simulink model "gm_final_heart_sym2_level4_hdl"  (R2021a)
settings: Solver=FixedStepDiscrete  StartTime=0.0  StopTime=8  RelTol=1e-3
libraries: hdlmdlgenlib x45
(part 3 of 3)

== system gm_final_heart_sym2_level4_hdl/DWT_Sym2_Level4/1st_Level_Recon2/LoR_Odd ==
  In_LoR_o : Inport  OutDataTypeStr=fixdt(1, 16, 23)  PortDimensions=1  SampleTime=2.26757369614512e-05
  Add : Sum  AccumDataTypeStr=fixdt(1, 16, 23)  OutDataTypeStr=fixdt(1, 16, 23)  SampleTime=2.26757369614512e-05
  Constant11 : Constant  Value=-0.1294097900390625  OutDataTypeStr=fixdt(1, 16, 17)  SampleTime=2.26757369614512e-05
  Constant9 : Constant  Value=0.836517333984375  OutDataTypeStr=fixdt(0, 16, 16)  SampleTime=2.26757369614512e-05
  Delay : Delay  DelayLength=double(1)  InitialCondition=0  SampleTime=2.26757369614512e-05
  HwModeRegister{,1..3} (4 alike) : Delay  DelayLength=double(1)  InitialCondition=0  SampleTime=2.26757369614512e-05
  Multiply : Product  Inputs=**  OutDataTypeStr=fixdt(1, 16, 23)  SampleTime=2.26757369614512e-05
  Multiply1 : Product  Inputs=**  OutDataTypeStr=fixdt(1, 16, 26)  SampleTime=2.26757369614512e-05
  PipelineRegister : Delay  DelayLength=double(1)  InitialCondition=0  SampleTime=2.26757369614512e-05
  PipelineRegister1 : Delay  DelayLength=double(1)  InitialCondition=0  SampleTime=2.26757369614512e-05
  Rate Transition : hdlmdlgenlib/Buffer
      settings: SourceProductBaseCode=SL
  delayMatch : Delay  DelayLength=double(1)  InitialCondition=0  SampleTime=2.26757369614512e-05
  Out_HiR_o : Outport  OutDataTypeStr=fixdt(1,16,23)  SampleTime=2.26757369614512e-05  VectorParamsAs1DForOutWhenUnconnected=off
  wires:
  Add/1 -> Out_HiR_o/1
  Constant11/1 -> HwModeRegister2/1
  Constant9/1 -> HwModeRegister/1
  Delay/1 -> Rate Transition/1
  PipelineRegister/1 -> Add/1
  delayMatch/1 -> Add/2
  Rate Transition/1 -> HwModeRegister3/1
  In_LoR_o/1 -> Delay/1, HwModeRegister1/1
  PipelineRegister1/1 -> delayMatch/1
  Multiply/1 -> PipelineRegister/1
  HwModeRegister/1 -> Multiply/1
  HwModeRegister1/1 -> Multiply/2
  Multiply1/1 -> PipelineRegister1/1
  HwModeRegister2/1 -> Multiply1/1
  HwModeRegister3/1 -> Multiply1/2

== system gm_final_heart_sym2_level4_hdl/DWT_Sym2_Level4/1st_Level_Recon3/HiR_Even ==
  In_HiR_e : Inport  OutDataTypeStr=fixdt(1, 16, 28)  PortDimensions=1  SampleTime=2.26757369614512e-05
  Add : Sum  AccumDataTypeStr=fixdt(1, 16, 28)  OutDataTypeStr=fixdt(1, 16, 28)  SampleTime=2.26757369614512e-05
  Constant12 : Constant  Value=-0.1294097900390625  OutDataTypeStr=fixdt(1, 16, 17)  SampleTime=2.26757369614512e-05
  Constant14 : Constant  Value=0.836517333984375  OutDataTypeStr=fixdt(0, 16, 16)  SampleTime=2.26757369614512e-05
  Delay : Delay  DelayLength=double(1)  InitialCondition=0  SampleTime=2.26757369614512e-05
  HwModeRegister{,1..3} (4 alike) : Delay  DelayLength=double(1)  InitialCondition=0  SampleTime=2.26757369614512e-05
  Multiply : Product  Inputs=**  OutDataTypeStr=fixdt(1, 16, 30)  SampleTime=2.26757369614512e-05
  Multiply1 : Product  Inputs=**  OutDataTypeStr=fixdt(1, 16, 28)  SampleTime=2.26757369614512e-05
  PipelineRegister : Delay  DelayLength=double(1)  InitialCondition=0  SampleTime=2.26757369614512e-05
  PipelineRegister1 : Delay  DelayLength=double(1)  InitialCondition=0  SampleTime=2.26757369614512e-05
  Rate Transition : hdlmdlgenlib/Buffer
      settings: SourceProductBaseCode=SL
  delayMatch : Delay  DelayLength=double(1)  InitialCondition=0  SampleTime=2.26757369614512e-05
  Out_HiR_e : Outport  OutDataTypeStr=fixdt(1,16,28)  SampleTime=2.26757369614512e-05  VectorParamsAs1DForOutWhenUnconnected=off
  wires:
  Add/1 -> Out_HiR_e/1
  Constant12/1 -> HwModeRegister/1
  Constant14/1 -> HwModeRegister2/1
  Delay/1 -> Rate Transition/1
  PipelineRegister/1 -> Add/1
  delayMatch/1 -> Add/2
  Rate Transition/1 -> HwModeRegister3/1
  In_HiR_e/1 -> Delay/1, HwModeRegister1/1
  PipelineRegister1/1 -> delayMatch/1
  Multiply/1 -> PipelineRegister/1
  HwModeRegister/1 -> Multiply/1
  HwModeRegister1/1 -> Multiply/2
  Multiply1/1 -> PipelineRegister1/1
  HwModeRegister2/1 -> Multiply1/1
  HwModeRegister3/1 -> Multiply1/2

== system gm_final_heart_sym2_level4_hdl/DWT_Sym2_Level4/1st_Level_Recon3/HiR_Odd ==
  In_HiR_o : Inport  OutDataTypeStr=fixdt(1, 16, 28)  PortDimensions=1  SampleTime=2.26757369614512e-05
  Add : Sum  AccumDataTypeStr=fixdt(1, 16, 28)  OutDataTypeStr=fixdt(1, 16, 28)  SampleTime=2.26757369614512e-05
  Constant13 : Constant  Value=-0.22414398193359375  OutDataTypeStr=fixdt(1, 16, 17)  SampleTime=2.26757369614512e-05
  Constant15 : Constant  Value=-0.4829559326171875  OutDataTypeStr=fixdt(1, 16, 16)  SampleTime=2.26757369614512e-05
  Delay : Delay  DelayLength=double(1)  InitialCondition=0  SampleTime=2.26757369614512e-05
  HwModeRegister{,1..3} (4 alike) : Delay  DelayLength=double(1)  InitialCondition=0  SampleTime=2.26757369614512e-05
  Multiply : Product  Inputs=**  OutDataTypeStr=fixdt(1, 16, 30)  SampleTime=2.26757369614512e-05
  Multiply1 : Product  Inputs=**  OutDataTypeStr=fixdt(1, 16, 29)  SampleTime=2.26757369614512e-05
  PipelineRegister : Delay  DelayLength=double(1)  InitialCondition=0  SampleTime=2.26757369614512e-05
  PipelineRegister1 : Delay  DelayLength=double(1)  InitialCondition=0  SampleTime=2.26757369614512e-05
  Rate Transition : hdlmdlgenlib/Buffer
      settings: SourceProductBaseCode=SL
  delayMatch : Delay  DelayLength=double(1)  InitialCondition=0  SampleTime=2.26757369614512e-05
  Out_HiR_o : Outport  OutDataTypeStr=fixdt(1,16,28)  SampleTime=2.26757369614512e-05  VectorParamsAs1DForOutWhenUnconnected=off
  wires:
  Add/1 -> Out_HiR_o/1
  Constant13/1 -> HwModeRegister/1
  Constant15/1 -> HwModeRegister2/1
  Delay/1 -> Rate Transition/1
  PipelineRegister/1 -> Add/1
  delayMatch/1 -> Add/2
  Rate Transition/1 -> HwModeRegister3/1
  In_HiR_o/1 -> Delay/1, HwModeRegister1/1
  PipelineRegister1/1 -> delayMatch/1
  Multiply/1 -> PipelineRegister/1
  HwModeRegister/1 -> Multiply/1
  HwModeRegister1/1 -> Multiply/2
  Multiply1/1 -> PipelineRegister1/1
  HwModeRegister2/1 -> Multiply1/1
  HwModeRegister3/1 -> Multiply1/2

== system gm_final_heart_sym2_level4_hdl/DWT_Sym2_Level4/1st_Level_Recon3/LoR_Even ==
  In_LoR_e : Inport  OutDataTypeStr=fixdt(1, 16, 22)  PortDimensions=1  SampleTime=2.26757369614512e-05
  Add : Sum  AccumDataTypeStr=fixdt(1, 16, 23)  OutDataTypeStr=fixdt(1, 16, 23)  SampleTime=2.26757369614512e-05
  Constant10 : Constant  Value=0.22414398193359375  OutDataTypeStr=fixdt(0, 16, 18)  SampleTime=2.26757369614512e-05
  Constant8 : Constant  Value=0.48296356201171875  OutDataTypeStr=fixdt(0, 16, 17)  SampleTime=2.26757369614512e-05
  Delay : Delay  DelayLength=double(1)  InitialCondition=0  SampleTime=2.26757369614512e-05
  HwModeRegister{,1..3} (4 alike) : Delay  DelayLength=double(1)  InitialCondition=0  SampleTime=2.26757369614512e-05
  Multiply : Product  Inputs=**  OutDataTypeStr=fixdt(1, 16, 23)  SampleTime=2.26757369614512e-05
  Multiply1 : Product  Inputs=**  OutDataTypeStr=fixdt(1, 16, 25)  SampleTime=2.26757369614512e-05
  PipelineRegister : Delay  DelayLength=double(1)  InitialCondition=0  SampleTime=2.26757369614512e-05
  PipelineRegister1 : Delay  DelayLength=double(1)  InitialCondition=0  SampleTime=2.26757369614512e-05
  Rate Transition : hdlmdlgenlib/Buffer
      settings: SourceProductBaseCode=SL
  delayMatch : Delay  DelayLength=double(1)  InitialCondition=0  SampleTime=2.26757369614512e-05
  Out_LoR_e : Outport  OutDataTypeStr=fixdt(1,16,23)  SampleTime=2.26757369614512e-05  VectorParamsAs1DForOutWhenUnconnected=off
  wires:
  Add/1 -> Out_LoR_e/1
  Constant10/1 -> HwModeRegister2/1
  Constant8/1 -> HwModeRegister/1
  Delay/1 -> Rate Transition/1
  PipelineRegister/1 -> Add/1
  delayMatch/1 -> Add/2
  Rate Transition/1 -> HwModeRegister3/1
  In_LoR_e/1 -> Delay/1, HwModeRegister1/1
  PipelineRegister1/1 -> delayMatch/1
  Multiply/1 -> PipelineRegister/1
  HwModeRegister/1 -> Multiply/1
  HwModeRegister1/1 -> Multiply/2
  Multiply1/1 -> PipelineRegister1/1
  HwModeRegister2/1 -> Multiply1/1
  HwModeRegister3/1 -> Multiply1/2

== system gm_final_heart_sym2_level4_hdl/DWT_Sym2_Level4/1st_Level_Recon3/LoR_Odd ==
  In_LoR_o : Inport  OutDataTypeStr=fixdt(1, 16, 22)  PortDimensions=1  SampleTime=2.26757369614512e-05
  Add : Sum  AccumDataTypeStr=fixdt(1, 16, 23)  OutDataTypeStr=fixdt(1, 16, 23)  SampleTime=2.26757369614512e-05
  Constant11 : Constant  Value=-0.1294097900390625  OutDataTypeStr=fixdt(1, 16, 17)  SampleTime=2.26757369614512e-05
  Constant9 : Constant  Value=0.836517333984375  OutDataTypeStr=fixdt(0, 16, 16)  SampleTime=2.26757369614512e-05
  Delay : Delay  DelayLength=double(1)  InitialCondition=0  SampleTime=2.26757369614512e-05
  HwModeRegister{,1..3} (4 alike) : Delay  DelayLength=double(1)  InitialCondition=0  SampleTime=2.26757369614512e-05
  Multiply : Product  Inputs=**  OutDataTypeStr=fixdt(1, 16, 23)  SampleTime=2.26757369614512e-05
  Multiply1 : Product  Inputs=**  OutDataTypeStr=fixdt(1, 16, 25)  SampleTime=2.26757369614512e-05
  PipelineRegister : Delay  DelayLength=double(1)  InitialCondition=0  SampleTime=2.26757369614512e-05
  PipelineRegister1 : Delay  DelayLength=double(1)  InitialCondition=0  SampleTime=2.26757369614512e-05
  Rate Transition : hdlmdlgenlib/Buffer
      settings: SourceProductBaseCode=SL
  delayMatch : Delay  DelayLength=double(1)  InitialCondition=0  SampleTime=2.26757369614512e-05
  Out_HiR_o : Outport  OutDataTypeStr=fixdt(1,16,23)  SampleTime=2.26757369614512e-05  VectorParamsAs1DForOutWhenUnconnected=off
  wires:
  Add/1 -> Out_HiR_o/1
  Constant11/1 -> HwModeRegister2/1
  Constant9/1 -> HwModeRegister/1
  Delay/1 -> Rate Transition/1
  PipelineRegister/1 -> Add/1
  delayMatch/1 -> Add/2
  Rate Transition/1 -> HwModeRegister3/1
  In_LoR_o/1 -> Delay/1, HwModeRegister1/1
  PipelineRegister1/1 -> delayMatch/1
  Multiply/1 -> PipelineRegister/1
  HwModeRegister/1 -> Multiply/1
  HwModeRegister1/1 -> Multiply/2
  Multiply1/1 -> PipelineRegister1/1
  HwModeRegister2/1 -> Multiply1/1
  HwModeRegister3/1 -> Multiply1/2

== system gm_final_heart_sym2_level4_hdl/DWT_Sym2_Level4/Threshold_Estimator/Absolute_Value1 ==
  Signal_w4 : Inport  OutDataTypeStr=fixdt(1, 16, 26)  PortDimensions=1  SampleTime=2.26757369614512e-05
  Absolute_Switch : Switch  Threshold=double(1)  OutDataTypeStr=fixdt(0, 16, 27)  SampleTime=2.26757369614512e-05
  Constant295 : Constant  Value=0  OutDataTypeStr=fixdt(1, 16, 4)  SampleTime=2.26757369614512e-05
  Gain2 : Product  Inputs=**  OutDataTypeStr=fixdt(0, 16, 28)  SampleTime=2.26757369614512e-05
  Gain2_const : Constant  Value=-1  OutDataTypeStr=fixdt(1, 16, 15)  SampleTime=2.26757369614512e-05
  HwModeRegister : Delay  DelayLength=double(1)  InitialCondition=0  SampleTime=2.26757369614512e-05
  HwModeRegister1 : Delay  DelayLength=double(1)  InitialCondition=0  SampleTime=2.26757369614512e-05
  PipelineRegister : Delay  DelayLength=double(1)  InitialCondition=0  SampleTime=2.26757369614512e-05
  Relational Operator2 : RelationalOperator  Operator=<  OutDataTypeStr=boolean  SampleTime=2.26757369614512e-05  RndMeth=Nearest
  delayMatch : Delay  DelayLength=double(2)  InitialCondition=0  SampleTime=2.26757369614512e-05
  delayMatch1 : Delay  DelayLength=double(2)  InitialCondition=0  SampleTime=2.26757369614512e-05
  Out_Abs : Outport  OutDataTypeStr=fixdt(0,16,27)  SampleTime=2.26757369614512e-05  VectorParamsAs1DForOutWhenUnconnected=off
  wires:
  delayMatch1/1 -> Absolute_Switch/3
  Absolute_Switch/1 -> Out_Abs/1
  Constant295/1 -> Relational Operator2/2
  PipelineRegister/1 -> Absolute_Switch/1
  delayMatch/1 -> Absolute_Switch/2
  Gain2_const/1 -> HwModeRegister/1
  Signal_w4/1 -> delayMatch1/1, Relational Operator2/1, HwModeRegister1/1
  Relational Operator2/1 -> delayMatch/1
  Gain2/1 -> PipelineRegister/1
  HwModeRegister/1 -> Gain2/1
  HwModeRegister1/1 -> Gain2/2

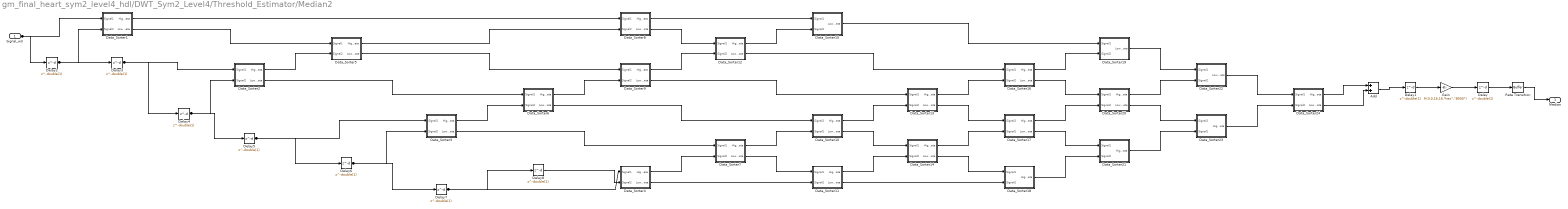
== system gm_final_heart_sym2_level4_hdl/DWT_Sym2_Level4/Threshold_Estimator/Median2 ==
  Signal_w3 : Inport  OutDataTypeStr=fixdt(0, 16, 27)  PortDimensions=1  SampleTime=2.26757369614512e-05
  Add : Sum  AccumDataTypeStr=fixdt(0, 16, 26)  OutDataTypeStr=fixdt(0, 16, 26)  SampleTime=2.26757369614512e-05
  Data_Sorter1 : Subsystem
  Data_Sorter10 : Subsystem
  Data_Sorter11 : Subsystem
  Data_Sorter12 : Subsystem
  Data_Sorter13 : Subsystem
  Data_Sorter14 : Subsystem
  Data_Sorter15 : Subsystem
  Data_Sorter16 : Subsystem
  Data_Sorter17 : Subsystem
  Data_Sorter18 : Subsystem
  Data_Sorter19 : Subsystem
  Data_Sorter2 : Subsystem
  Data_Sorter20 : Subsystem
  Data_Sorter21 : Subsystem
  Data_Sorter22 : Subsystem
  Data_Sorter23 : Subsystem
  Data_Sorter24 : Subsystem
  Data_Sorter3 : Subsystem
  Data_Sorter4 : Subsystem
  Data_Sorter5 : Subsystem
  Data_Sorter6 : Subsystem
  Data_Sorter7 : Subsystem
  Data_Sorter8 : Subsystem
  Data_Sorter9 : Subsystem
  Delay{,1..8} (9 alike) : Delay  DelayLength=double(1)  InitialCondition=0  SampleTime=2.26757369614512e-05
  Gain : Gain  Gain="fi(0,0,16,16,\"hex\",\"8000\")"  ParamDataTypeStr=fixdt(0, 16, 16)  OutDataTypeStr=fixdt(0, 16, 27)  SampleTime=2.26757369614512e-05
  Rate Transition : hdlmdlgenlib/Buffer
      settings: SourceProductBaseCode=SL
  Median : Outport  OutDataTypeStr=fixdt(0,16,27)  SampleTime=2.26757369614512e-05  VectorParamsAs1DForOutWhenUnconnected=off
  wires:
  Add/1 -> Delay1/1
  Data_Sorter1/1(High_Data) -> Data_Sorter8/1(Signal1)
  Data_Sorter1/2(Low_Data) -> Data_Sorter5/1(Signal1)
  Data_Sorter10/1(High_Data) -> Data_Sorter13/2(Signal2)
  Data_Sorter10/2(Low_Data) -> Data_Sorter14/1(Signal1)
  Data_Sorter11/1(High_Data) -> Data_Sorter14/2(Signal2)
  Data_Sorter11/2(Low_Data) -> Data_Sorter18/2(Signal2)
  Data_Sorter12/1(High_Data) -> Data_Sorter15/2(Signal2)
  Data_Sorter12/2(Low_Data) -> Data_Sorter16/1(Signal1)
  Data_Sorter13/1(High_Data) -> Data_Sorter16/2(Signal2)
  Data_Sorter13/2(Low_Data) -> Data_Sorter17/1(Signal1)
  Data_Sorter14/1(High_Data) -> Data_Sorter17/2(Signal2)
  Data_Sorter14/2(Low_Data) -> Data_Sorter18/1(Signal1)
  Data_Sorter15/1(Low_Data) -> Data_Sorter19/1(Signal1)
  Data_Sorter16/1(High_Data) -> Data_Sorter19/2(Signal2)
  Data_Sorter16/2(Low_Data) -> Data_Sorter20/1(Signal1)
  Data_Sorter17/1(High_Data) -> Data_Sorter20/2(Signal2)
  Data_Sorter17/2(Low_Data) -> Data_Sorter21/1(Signal1)
  Data_Sorter18/1(High_Data) -> Data_Sorter21/2(Signal2)
  Data_Sorter19/1(Low_Data) -> Data_Sorter22/1(Signal1)
  Data_Sorter2/1(High_Data) -> Data_Sorter5/2(Signal2)
  Data_Sorter2/2(Low_Data) -> Data_Sorter6/1(Signal1)
  Data_Sorter20/1(High_Data) -> Data_Sorter22/2(Signal2)
  Data_Sorter20/2(Low_Data) -> Data_Sorter23/1(Signal1)
  Data_Sorter21/1(High_Data) -> Data_Sorter23/2(Signal2)
  Data_Sorter22/1(Low_Data) -> Data_Sorter24/1(Signal1)
  Data_Sorter23/1(High_Data) -> Data_Sorter24/2(Signal2)
  Data_Sorter24/1(High_Data) -> Add/1
  Data_Sorter24/2(Low_Data) -> Add/2
  Data_Sorter3/1(High_Data) -> Data_Sorter6/2(Signal2)
  Data_Sorter3/2(Low_Data) -> Data_Sorter7/1(Signal1)
  Data_Sorter4/1(High_Data) -> Data_Sorter7/2(Signal2)
  Data_Sorter4/2(Low_Data) -> Data_Sorter11/2(Signal2)
  Data_Sorter5/1(High_Data) -> Data_Sorter8/2(Signal2)
  Data_Sorter5/2(Low_Data) -> Data_Sorter9/1(Signal1)
  Data_Sorter6/1(High_Data) -> Data_Sorter9/2(Signal2)
  Data_Sorter6/2(Low_Data) -> Data_Sorter10/1(Signal1)
  Data_Sorter7/1(High_Data) -> Data_Sorter10/2(Signal2)
  Data_Sorter7/2(Low_Data) -> Data_Sorter11/1(Signal1)
  Data_Sorter8/1(High_Data) -> Data_Sorter15/1(Signal1)
  Data_Sorter8/2(Low_Data) -> Data_Sorter12/1(Signal1)
  Data_Sorter9/1(High_Data) -> Data_Sorter12/2(Signal2)
  Data_Sorter9/2(Low_Data) -> Data_Sorter13/1(Signal1)
  Delay/1 -> Rate Transition/1
  Delay1/1 -> Gain/1
  Delay2/1 -> Delay3/1, Data_Sorter1/2(Signal2)
  Delay3/1 -> Delay4/1, Data_Sorter2/1(Signal1)
  Delay4/1 -> Delay5/1, Data_Sorter2/2(Signal2)
  Delay5/1 -> Delay6/1, Data_Sorter3/1(Signal1)
  Delay6/1 -> Delay7/1, Data_Sorter3/2(Signal2)
  Delay7/1 -> Delay8/1, Data_Sorter4/1(Signal1)
  Delay8/1 -> Data_Sorter4/2(Signal2)
  Gain/1 -> Delay/1
  Rate Transition/1 -> Median/1
  Signal_w3/1 -> Delay2/1, Data_Sorter1/1(Signal1)

== system gm_final_heart_sym2_level4_hdl/DWT_Sym2_Level4/Threshold_Estimator/Median2/Data_Sorter1 ==
  Signal1 : Inport  OutDataTypeStr=fixdt(0, 16, 27)  PortDimensions=1  SampleTime=2.26757369614512e-05
  Signal2 : Inport  Port=2  OutDataTypeStr=fixdt(0, 16, 27)  PortDimensions=1  SampleTime=2.26757369614512e-05
  Data_Sorter_Switch : Switch  Criteria=u2 ~= 0  Threshold=double(0)  OutDataTypeStr=fixdt(0, 16, 27)  SampleTime=2.26757369614512e-05
  Data_Sorter_Switch1 : Switch  Threshold=double(1)  OutDataTypeStr=fixdt(0, 16, 27)  SampleTime=2.26757369614512e-05
  Delay1 : Delay  DelayLength=double(1)  InitialCondition=0  SampleTime=2.26757369614512e-05
  Delay2 : Delay  DelayLength=double(1)  InitialCondition=0  SampleTime=2.26757369614512e-05
  Relational Operator2 : RelationalOperator  Operator=<  OutDataTypeStr=boolean  SampleTime=2.26757369614512e-05  RndMeth=Nearest
  High_Data : Outport  OutDataTypeStr=fixdt(0,16,27)  SampleTime=2.26757369614512e-05  VectorParamsAs1DForOutWhenUnconnected=off
  Low_Data : Outport  Port=2  OutDataTypeStr=fixdt(0,16,27)  SampleTime=2.26757369614512e-05  VectorParamsAs1DForOutWhenUnconnected=off
  wires:
  Data_Sorter_Switch/1 -> Delay1/1
  Data_Sorter_Switch1/1 -> Delay2/1
  Delay1/1 -> High_Data/1
  Delay2/1 -> Low_Data/1
  Relational Operator2/1 -> Data_Sorter_Switch1/2, Data_Sorter_Switch/2
  Signal1/1 -> Relational Operator2/1, Data_Sorter_Switch/3, Data_Sorter_Switch/1
  Signal2/1 -> Relational Operator2/2, Data_Sorter_Switch1/3, Data_Sorter_Switch1/1

== system gm_final_heart_sym2_level4_hdl/DWT_Sym2_Level4/Threshold_Estimator/Median2/Data_Sorter10 ==
  Signal1 : Inport  OutDataTypeStr=fixdt(0, 16, 27)  PortDimensions=1  SampleTime=2.26757369614512e-05
  Signal2 : Inport  Port=2  OutDataTypeStr=fixdt(0, 16, 27)  PortDimensions=1  SampleTime=2.26757369614512e-05
  Data_Sorter_Switch : Switch  Criteria=u2 ~= 0  Threshold=double(0)  OutDataTypeStr=fixdt(0, 16, 27)  SampleTime=2.26757369614512e-05
  Data_Sorter_Switch1 : Switch  Threshold=double(1)  OutDataTypeStr=fixdt(0, 16, 27)  SampleTime=2.26757369614512e-05
  Delay1 : Delay  DelayLength=double(1)  InitialCondition=0  SampleTime=2.26757369614512e-05
  Delay2 : Delay  DelayLength=double(1)  InitialCondition=0  SampleTime=2.26757369614512e-05
  Relational Operator2 : RelationalOperator  Operator=<  OutDataTypeStr=boolean  SampleTime=2.26757369614512e-05  RndMeth=Nearest
  High_Data : Outport  OutDataTypeStr=fixdt(0,16,27)  SampleTime=2.26757369614512e-05  VectorParamsAs1DForOutWhenUnconnected=off
  Low_Data : Outport  Port=2  OutDataTypeStr=fixdt(0,16,27)  SampleTime=2.26757369614512e-05  VectorParamsAs1DForOutWhenUnconnected=off
  wires:
  Data_Sorter_Switch/1 -> Delay1/1
  Data_Sorter_Switch1/1 -> Delay2/1
  Delay1/1 -> High_Data/1
  Delay2/1 -> Low_Data/1
  Relational Operator2/1 -> Data_Sorter_Switch1/2, Data_Sorter_Switch/2
  Signal1/1 -> Relational Operator2/1, Data_Sorter_Switch/3, Data_Sorter_Switch/1
  Signal2/1 -> Relational Operator2/2, Data_Sorter_Switch1/3, Data_Sorter_Switch1/1

== system gm_final_heart_sym2_level4_hdl/DWT_Sym2_Level4/Threshold_Estimator/Median2/Data_Sorter11 ==
  Signal1 : Inport  OutDataTypeStr=fixdt(0, 16, 27)  PortDimensions=1  SampleTime=2.26757369614512e-05
  Signal2 : Inport  Port=2  OutDataTypeStr=fixdt(0, 16, 27)  PortDimensions=1  SampleTime=2.26757369614512e-05
  Data_Sorter_Switch : Switch  Criteria=u2 ~= 0  Threshold=double(0)  OutDataTypeStr=fixdt(0, 16, 27)  SampleTime=2.26757369614512e-05
  Data_Sorter_Switch1 : Switch  Threshold=double(1)  OutDataTypeStr=fixdt(0, 16, 27)  SampleTime=2.26757369614512e-05
  Delay1 : Delay  DelayLength=double(1)  InitialCondition=0  SampleTime=2.26757369614512e-05
  Delay2 : Delay  DelayLength=double(1)  InitialCondition=0  SampleTime=2.26757369614512e-05
  Relational Operator2 : RelationalOperator  Operator=<  OutDataTypeStr=boolean  SampleTime=2.26757369614512e-05  RndMeth=Nearest
  High_Data : Outport  OutDataTypeStr=fixdt(0,16,27)  SampleTime=2.26757369614512e-05  VectorParamsAs1DForOutWhenUnconnected=off
  Low_Data : Outport  Port=2  OutDataTypeStr=fixdt(0,16,27)  SampleTime=2.26757369614512e-05  VectorParamsAs1DForOutWhenUnconnected=off
  wires:
  Data_Sorter_Switch/1 -> Delay1/1
  Data_Sorter_Switch1/1 -> Delay2/1
  Delay1/1 -> High_Data/1
  Delay2/1 -> Low_Data/1
  Relational Operator2/1 -> Data_Sorter_Switch1/2, Data_Sorter_Switch/2
  Signal1/1 -> Relational Operator2/1, Data_Sorter_Switch/3, Data_Sorter_Switch/1
  Signal2/1 -> Relational Operator2/2, Data_Sorter_Switch1/3, Data_Sorter_Switch1/1

== system gm_final_heart_sym2_level4_hdl/DWT_Sym2_Level4/Threshold_Estimator/Median2/Data_Sorter12 ==
  Signal1 : Inport  OutDataTypeStr=fixdt(0, 16, 27)  PortDimensions=1  SampleTime=2.26757369614512e-05
  Signal2 : Inport  Port=2  OutDataTypeStr=fixdt(0, 16, 27)  PortDimensions=1  SampleTime=2.26757369614512e-05
  Data_Sorter_Switch : Switch  Criteria=u2 ~= 0  Threshold=double(0)  OutDataTypeStr=fixdt(0, 16, 27)  SampleTime=2.26757369614512e-05
  Data_Sorter_Switch1 : Switch  Threshold=double(1)  OutDataTypeStr=fixdt(0, 16, 27)  SampleTime=2.26757369614512e-05
  Delay1 : Delay  DelayLength=double(1)  InitialCondition=0  SampleTime=2.26757369614512e-05
  Delay2 : Delay  DelayLength=double(1)  InitialCondition=0  SampleTime=2.26757369614512e-05
  Relational Operator2 : RelationalOperator  Operator=<  OutDataTypeStr=boolean  SampleTime=2.26757369614512e-05  RndMeth=Nearest
  High_Data : Outport  OutDataTypeStr=fixdt(0,16,27)  SampleTime=2.26757369614512e-05  VectorParamsAs1DForOutWhenUnconnected=off
  Low_Data : Outport  Port=2  OutDataTypeStr=fixdt(0,16,27)  SampleTime=2.26757369614512e-05  VectorParamsAs1DForOutWhenUnconnected=off
  wires:
  Data_Sorter_Switch/1 -> Delay1/1
  Data_Sorter_Switch1/1 -> Delay2/1
  Delay1/1 -> High_Data/1
  Delay2/1 -> Low_Data/1
  Relational Operator2/1 -> Data_Sorter_Switch1/2, Data_Sorter_Switch/2
  Signal1/1 -> Relational Operator2/1, Data_Sorter_Switch/3, Data_Sorter_Switch/1
  Signal2/1 -> Relational Operator2/2, Data_Sorter_Switch1/3, Data_Sorter_Switch1/1

== system gm_final_heart_sym2_level4_hdl/DWT_Sym2_Level4/Threshold_Estimator/Median2/Data_Sorter13 ==
  Signal1 : Inport  OutDataTypeStr=fixdt(0, 16, 27)  PortDimensions=1  SampleTime=2.26757369614512e-05
  Signal2 : Inport  Port=2  OutDataTypeStr=fixdt(0, 16, 27)  PortDimensions=1  SampleTime=2.26757369614512e-05
  Data_Sorter_Switch : Switch  Criteria=u2 ~= 0  Threshold=double(0)  OutDataTypeStr=fixdt(0, 16, 27)  SampleTime=2.26757369614512e-05
  Data_Sorter_Switch1 : Switch  Threshold=double(1)  OutDataTypeStr=fixdt(0, 16, 27)  SampleTime=2.26757369614512e-05
  Delay1 : Delay  DelayLength=double(1)  InitialCondition=0  SampleTime=2.26757369614512e-05
  Delay2 : Delay  DelayLength=double(1)  InitialCondition=0  SampleTime=2.26757369614512e-05
  Relational Operator2 : RelationalOperator  Operator=<  OutDataTypeStr=boolean  SampleTime=2.26757369614512e-05  RndMeth=Nearest
  High_Data : Outport  OutDataTypeStr=fixdt(0,16,27)  SampleTime=2.26757369614512e-05  VectorParamsAs1DForOutWhenUnconnected=off
  Low_Data : Outport  Port=2  OutDataTypeStr=fixdt(0,16,27)  SampleTime=2.26757369614512e-05  VectorParamsAs1DForOutWhenUnconnected=off
  wires:
  Data_Sorter_Switch/1 -> Delay1/1
  Data_Sorter_Switch1/1 -> Delay2/1
  Delay1/1 -> High_Data/1
  Delay2/1 -> Low_Data/1
  Relational Operator2/1 -> Data_Sorter_Switch1/2, Data_Sorter_Switch/2
  Signal1/1 -> Relational Operator2/1, Data_Sorter_Switch/3, Data_Sorter_Switch/1
  Signal2/1 -> Relational Operator2/2, Data_Sorter_Switch1/3, Data_Sorter_Switch1/1

== system gm_final_heart_sym2_level4_hdl/DWT_Sym2_Level4/Threshold_Estimator/Median2/Data_Sorter14 ==
  Signal1 : Inport  OutDataTypeStr=fixdt(0, 16, 27)  PortDimensions=1  SampleTime=2.26757369614512e-05
  Signal2 : Inport  Port=2  OutDataTypeStr=fixdt(0, 16, 27)  PortDimensions=1  SampleTime=2.26757369614512e-05
  Data_Sorter_Switch : Switch  Criteria=u2 ~= 0  Threshold=double(0)  OutDataTypeStr=fixdt(0, 16, 27)  SampleTime=2.26757369614512e-05
  Data_Sorter_Switch1 : Switch  Threshold=double(1)  OutDataTypeStr=fixdt(0, 16, 27)  SampleTime=2.26757369614512e-05
  Delay1 : Delay  DelayLength=double(1)  InitialCondition=0  SampleTime=2.26757369614512e-05
  Delay2 : Delay  DelayLength=double(1)  InitialCondition=0  SampleTime=2.26757369614512e-05
  Relational Operator2 : RelationalOperator  Operator=<  OutDataTypeStr=boolean  SampleTime=2.26757369614512e-05  RndMeth=Nearest
  High_Data : Outport  OutDataTypeStr=fixdt(0,16,27)  SampleTime=2.26757369614512e-05  VectorParamsAs1DForOutWhenUnconnected=off
  Low_Data : Outport  Port=2  OutDataTypeStr=fixdt(0,16,27)  SampleTime=2.26757369614512e-05  VectorParamsAs1DForOutWhenUnconnected=off
  wires:
  Data_Sorter_Switch/1 -> Delay1/1
  Data_Sorter_Switch1/1 -> Delay2/1
  Delay1/1 -> High_Data/1
  Delay2/1 -> Low_Data/1
  Relational Operator2/1 -> Data_Sorter_Switch1/2, Data_Sorter_Switch/2
  Signal1/1 -> Relational Operator2/1, Data_Sorter_Switch/3, Data_Sorter_Switch/1
  Signal2/1 -> Relational Operator2/2, Data_Sorter_Switch1/3, Data_Sorter_Switch1/1

== system gm_final_heart_sym2_level4_hdl/DWT_Sym2_Level4/Threshold_Estimator/Median2/Data_Sorter15 ==
  Signal1 : Inport  OutDataTypeStr=fixdt(0, 16, 27)  PortDimensions=1  SampleTime=2.26757369614512e-05
  Signal2 : Inport  Port=2  OutDataTypeStr=fixdt(0, 16, 27)  PortDimensions=1  SampleTime=2.26757369614512e-05
  Data_Sorter_Switch1 : Switch  Threshold=double(1)  OutDataTypeStr=fixdt(0, 16, 27)  SampleTime=2.26757369614512e-05
  Delay2 : Delay  DelayLength=double(1)  InitialCondition=0  SampleTime=2.26757369614512e-05
  Relational Operator2 : RelationalOperator  Operator=<  OutDataTypeStr=boolean  SampleTime=2.26757369614512e-05  RndMeth=Nearest
  Low_Data : Outport  OutDataTypeStr=fixdt(0,16,27)  SampleTime=2.26757369614512e-05  VectorParamsAs1DForOutWhenUnconnected=off
  wires:
  Data_Sorter_Switch1/1 -> Delay2/1
  Delay2/1 -> Low_Data/1
  Relational Operator2/1 -> Data_Sorter_Switch1/2
  Signal1/1 -> Relational Operator2/1
  Signal2/1 -> Relational Operator2/2, Data_Sorter_Switch1/3, Data_Sorter_Switch1/1

== system gm_final_heart_sym2_level4_hdl/DWT_Sym2_Level4/Threshold_Estimator/Median2/Data_Sorter16 ==
  Signal1 : Inport  OutDataTypeStr=fixdt(0, 16, 27)  PortDimensions=1  SampleTime=2.26757369614512e-05
  Signal2 : Inport  Port=2  OutDataTypeStr=fixdt(0, 16, 27)  PortDimensions=1  SampleTime=2.26757369614512e-05
  Data_Sorter_Switch : Switch  Criteria=u2 ~= 0  Threshold=double(0)  OutDataTypeStr=fixdt(0, 16, 27)  SampleTime=2.26757369614512e-05
  Data_Sorter_Switch1 : Switch  Threshold=double(1)  OutDataTypeStr=fixdt(0, 16, 27)  SampleTime=2.26757369614512e-05
  Delay1 : Delay  DelayLength=double(1)  InitialCondition=0  SampleTime=2.26757369614512e-05
  Delay2 : Delay  DelayLength=double(1)  InitialCondition=0  SampleTime=2.26757369614512e-05
  Relational Operator2 : RelationalOperator  Operator=<  OutDataTypeStr=boolean  SampleTime=2.26757369614512e-05  RndMeth=Nearest
  High_Data : Outport  OutDataTypeStr=fixdt(0,16,27)  SampleTime=2.26757369614512e-05  VectorParamsAs1DForOutWhenUnconnected=off
  Low_Data : Outport  Port=2  OutDataTypeStr=fixdt(0,16,27)  SampleTime=2.26757369614512e-05  VectorParamsAs1DForOutWhenUnconnected=off
  wires:
  Data_Sorter_Switch/1 -> Delay1/1
  Data_Sorter_Switch1/1 -> Delay2/1
  Delay1/1 -> High_Data/1
  Delay2/1 -> Low_Data/1
  Relational Operator2/1 -> Data_Sorter_Switch1/2, Data_Sorter_Switch/2
  Signal1/1 -> Relational Operator2/1, Data_Sorter_Switch/3, Data_Sorter_Switch/1
  Signal2/1 -> Relational Operator2/2, Data_Sorter_Switch1/3, Data_Sorter_Switch1/1

== system gm_final_heart_sym2_level4_hdl/DWT_Sym2_Level4/Threshold_Estimator/Median2/Data_Sorter17 ==
  Signal1 : Inport  OutDataTypeStr=fixdt(0, 16, 27)  PortDimensions=1  SampleTime=2.26757369614512e-05
  Signal2 : Inport  Port=2  OutDataTypeStr=fixdt(0, 16, 27)  PortDimensions=1  SampleTime=2.26757369614512e-05
  Data_Sorter_Switch : Switch  Criteria=u2 ~= 0  Threshold=double(0)  OutDataTypeStr=fixdt(0, 16, 27)  SampleTime=2.26757369614512e-05
  Data_Sorter_Switch1 : Switch  Threshold=double(1)  OutDataTypeStr=fixdt(0, 16, 27)  SampleTime=2.26757369614512e-05
  Delay1 : Delay  DelayLength=double(1)  InitialCondition=0  SampleTime=2.26757369614512e-05
  Delay2 : Delay  DelayLength=double(1)  InitialCondition=0  SampleTime=2.26757369614512e-05
  Relational Operator2 : RelationalOperator  Operator=<  OutDataTypeStr=boolean  SampleTime=2.26757369614512e-05  RndMeth=Nearest
  High_Data : Outport  OutDataTypeStr=fixdt(0,16,27)  SampleTime=2.26757369614512e-05  VectorParamsAs1DForOutWhenUnconnected=off
  Low_Data : Outport  Port=2  OutDataTypeStr=fixdt(0,16,27)  SampleTime=2.26757369614512e-05  VectorParamsAs1DForOutWhenUnconnected=off
  wires:
  Data_Sorter_Switch/1 -> Delay1/1
  Data_Sorter_Switch1/1 -> Delay2/1
  Delay1/1 -> High_Data/1
  Delay2/1 -> Low_Data/1
  Relational Operator2/1 -> Data_Sorter_Switch1/2, Data_Sorter_Switch/2
  Signal1/1 -> Relational Operator2/1, Data_Sorter_Switch/3, Data_Sorter_Switch/1
  Signal2/1 -> Relational Operator2/2, Data_Sorter_Switch1/3, Data_Sorter_Switch1/1

== system gm_final_heart_sym2_level4_hdl/DWT_Sym2_Level4/Threshold_Estimator/Median2/Data_Sorter18 ==
  Signal1 : Inport  OutDataTypeStr=fixdt(0, 16, 27)  PortDimensions=1  SampleTime=2.26757369614512e-05
  Signal2 : Inport  Port=2  OutDataTypeStr=fixdt(0, 16, 27)  PortDimensions=1  SampleTime=2.26757369614512e-05
  Data_Sorter_Switch : Switch  Criteria=u2 ~= 0  Threshold=double(0)  OutDataTypeStr=fixdt(0, 16, 27)  SampleTime=2.26757369614512e-05
  Delay1 : Delay  DelayLength=double(1)  InitialCondition=0  SampleTime=2.26757369614512e-05
  Relational Operator2 : RelationalOperator  Operator=<  OutDataTypeStr=boolean  SampleTime=2.26757369614512e-05  RndMeth=Nearest
  High_Data : Outport  OutDataTypeStr=fixdt(0,16,27)  SampleTime=2.26757369614512e-05  VectorParamsAs1DForOutWhenUnconnected=off
  wires:
  Data_Sorter_Switch/1 -> Delay1/1
  Delay1/1 -> High_Data/1
  Relational Operator2/1 -> Data_Sorter_Switch/2
  Signal1/1 -> Relational Operator2/1, Data_Sorter_Switch/3, Data_Sorter_Switch/1
  Signal2/1 -> Relational Operator2/2

== system gm_final_heart_sym2_level4_hdl/DWT_Sym2_Level4/Threshold_Estimator/Median2/Data_Sorter19 ==
  Signal1 : Inport  OutDataTypeStr=fixdt(0, 16, 27)  PortDimensions=1  SampleTime=2.26757369614512e-05
  Signal2 : Inport  Port=2  OutDataTypeStr=fixdt(0, 16, 27)  PortDimensions=1  SampleTime=2.26757369614512e-05
  Data_Sorter_Switch1 : Switch  Threshold=double(1)  OutDataTypeStr=fixdt(0, 16, 27)  SampleTime=2.26757369614512e-05
  Delay2 : Delay  DelayLength=double(1)  InitialCondition=0  SampleTime=2.26757369614512e-05
  Relational Operator2 : RelationalOperator  Operator=<  OutDataTypeStr=boolean  SampleTime=2.26757369614512e-05  RndMeth=Nearest
  Low_Data : Outport  OutDataTypeStr=fixdt(0,16,27)  SampleTime=2.26757369614512e-05  VectorParamsAs1DForOutWhenUnconnected=off
  wires:
  Data_Sorter_Switch1/1 -> Delay2/1
  Delay2/1 -> Low_Data/1
  Relational Operator2/1 -> Data_Sorter_Switch1/2
  Signal1/1 -> Relational Operator2/1
  Signal2/1 -> Relational Operator2/2, Data_Sorter_Switch1/3, Data_Sorter_Switch1/1

== system gm_final_heart_sym2_level4_hdl/DWT_Sym2_Level4/Threshold_Estimator/Median2/Data_Sorter2 ==
  Signal1 : Inport  OutDataTypeStr=fixdt(0, 16, 27)  PortDimensions=1  SampleTime=2.26757369614512e-05
  Signal2 : Inport  Port=2  OutDataTypeStr=fixdt(0, 16, 27)  PortDimensions=1  SampleTime=2.26757369614512e-05
  Data_Sorter_Switch : Switch  Criteria=u2 ~= 0  Threshold=double(0)  OutDataTypeStr=fixdt(0, 16, 27)  SampleTime=2.26757369614512e-05
  Data_Sorter_Switch1 : Switch  Threshold=double(1)  OutDataTypeStr=fixdt(0, 16, 27)  SampleTime=2.26757369614512e-05
  Delay1 : Delay  DelayLength=double(1)  InitialCondition=0  SampleTime=2.26757369614512e-05
  Delay2 : Delay  DelayLength=double(1)  InitialCondition=0  SampleTime=2.26757369614512e-05
  Relational Operator2 : RelationalOperator  Operator=<  OutDataTypeStr=boolean  SampleTime=2.26757369614512e-05  RndMeth=Nearest
  High_Data : Outport  OutDataTypeStr=fixdt(0,16,27)  SampleTime=2.26757369614512e-05  VectorParamsAs1DForOutWhenUnconnected=off
  Low_Data : Outport  Port=2  OutDataTypeStr=fixdt(0,16,27)  SampleTime=2.26757369614512e-05  VectorParamsAs1DForOutWhenUnconnected=off
  wires:
  Data_Sorter_Switch/1 -> Delay1/1
  Data_Sorter_Switch1/1 -> Delay2/1
  Delay1/1 -> High_Data/1
  Delay2/1 -> Low_Data/1
  Relational Operator2/1 -> Data_Sorter_Switch1/2, Data_Sorter_Switch/2
  Signal1/1 -> Relational Operator2/1, Data_Sorter_Switch/3, Data_Sorter_Switch/1
  Signal2/1 -> Relational Operator2/2, Data_Sorter_Switch1/3, Data_Sorter_Switch1/1

== system gm_final_heart_sym2_level4_hdl/DWT_Sym2_Level4/Threshold_Estimator/Median2/Data_Sorter20 ==
  Signal1 : Inport  OutDataTypeStr=fixdt(0, 16, 27)  PortDimensions=1  SampleTime=2.26757369614512e-05
  Signal2 : Inport  Port=2  OutDataTypeStr=fixdt(0, 16, 27)  PortDimensions=1  SampleTime=2.26757369614512e-05
  Data_Sorter_Switch : Switch  Criteria=u2 ~= 0  Threshold=double(0)  OutDataTypeStr=fixdt(0, 16, 27)  SampleTime=2.26757369614512e-05
  Data_Sorter_Switch1 : Switch  Threshold=double(1)  OutDataTypeStr=fixdt(0, 16, 27)  SampleTime=2.26757369614512e-05
  Delay1 : Delay  DelayLength=double(1)  InitialCondition=0  SampleTime=2.26757369614512e-05
  Delay2 : Delay  DelayLength=double(1)  InitialCondition=0  SampleTime=2.26757369614512e-05
  Relational Operator2 : RelationalOperator  Operator=<  OutDataTypeStr=boolean  SampleTime=2.26757369614512e-05  RndMeth=Nearest
  High_Data : Outport  OutDataTypeStr=fixdt(0,16,27)  SampleTime=2.26757369614512e-05  VectorParamsAs1DForOutWhenUnconnected=off
  Low_Data : Outport  Port=2  OutDataTypeStr=fixdt(0,16,27)  SampleTime=2.26757369614512e-05  VectorParamsAs1DForOutWhenUnconnected=off
  wires:
  Data_Sorter_Switch/1 -> Delay1/1
  Data_Sorter_Switch1/1 -> Delay2/1
  Delay1/1 -> High_Data/1
  Delay2/1 -> Low_Data/1
  Relational Operator2/1 -> Data_Sorter_Switch1/2, Data_Sorter_Switch/2
  Signal1/1 -> Relational Operator2/1, Data_Sorter_Switch/3, Data_Sorter_Switch/1
  Signal2/1 -> Relational Operator2/2, Data_Sorter_Switch1/3, Data_Sorter_Switch1/1

== system gm_final_heart_sym2_level4_hdl/DWT_Sym2_Level4/Threshold_Estimator/Median2/Data_Sorter21 ==
  Signal1 : Inport  OutDataTypeStr=fixdt(0, 16, 27)  PortDimensions=1  SampleTime=2.26757369614512e-05
  Signal2 : Inport  Port=2  OutDataTypeStr=fixdt(0, 16, 27)  PortDimensions=1  SampleTime=2.26757369614512e-05
  Data_Sorter_Switch : Switch  Criteria=u2 ~= 0  Threshold=double(0)  OutDataTypeStr=fixdt(0, 16, 27)  SampleTime=2.26757369614512e-05
  Delay1 : Delay  DelayLength=double(1)  InitialCondition=0  SampleTime=2.26757369614512e-05
  Relational Operator2 : RelationalOperator  Operator=<  OutDataTypeStr=boolean  SampleTime=2.26757369614512e-05  RndMeth=Nearest
  High_Data : Outport  OutDataTypeStr=fixdt(0,16,27)  SampleTime=2.26757369614512e-05  VectorParamsAs1DForOutWhenUnconnected=off
  wires:
  Data_Sorter_Switch/1 -> Delay1/1
  Delay1/1 -> High_Data/1
  Relational Operator2/1 -> Data_Sorter_Switch/2
  Signal1/1 -> Relational Operator2/1, Data_Sorter_Switch/3, Data_Sorter_Switch/1
  Signal2/1 -> Relational Operator2/2

== system gm_final_heart_sym2_level4_hdl/DWT_Sym2_Level4/Threshold_Estimator/Median2/Data_Sorter22 ==
  Signal1 : Inport  OutDataTypeStr=fixdt(0, 16, 27)  PortDimensions=1  SampleTime=2.26757369614512e-05
  Signal2 : Inport  Port=2  OutDataTypeStr=fixdt(0, 16, 27)  PortDimensions=1  SampleTime=2.26757369614512e-05
  Data_Sorter_Switch1 : Switch  Threshold=double(1)  OutDataTypeStr=fixdt(0, 16, 27)  SampleTime=2.26757369614512e-05
  Delay2 : Delay  DelayLength=double(1)  InitialCondition=0  SampleTime=2.26757369614512e-05
  Relational Operator2 : RelationalOperator  Operator=<  OutDataTypeStr=boolean  SampleTime=2.26757369614512e-05  RndMeth=Nearest
  Low_Data : Outport  OutDataTypeStr=fixdt(0,16,27)  SampleTime=2.26757369614512e-05  VectorParamsAs1DForOutWhenUnconnected=off
  wires:
  Data_Sorter_Switch1/1 -> Delay2/1
  Delay2/1 -> Low_Data/1
  Relational Operator2/1 -> Data_Sorter_Switch1/2
  Signal1/1 -> Relational Operator2/1
  Signal2/1 -> Relational Operator2/2, Data_Sorter_Switch1/3, Data_Sorter_Switch1/1

== system gm_final_heart_sym2_level4_hdl/DWT_Sym2_Level4/Threshold_Estimator/Median2/Data_Sorter23 ==
  Signal1 : Inport  OutDataTypeStr=fixdt(0, 16, 27)  PortDimensions=1  SampleTime=2.26757369614512e-05
  Signal2 : Inport  Port=2  OutDataTypeStr=fixdt(0, 16, 27)  PortDimensions=1  SampleTime=2.26757369614512e-05
  Data_Sorter_Switch : Switch  Criteria=u2 ~= 0  Threshold=double(0)  OutDataTypeStr=fixdt(0, 16, 27)  SampleTime=2.26757369614512e-05
  Delay1 : Delay  DelayLength=double(1)  InitialCondition=0  SampleTime=2.26757369614512e-05
  Relational Operator2 : RelationalOperator  Operator=<  OutDataTypeStr=boolean  SampleTime=2.26757369614512e-05  RndMeth=Nearest
  High_Data : Outport  OutDataTypeStr=fixdt(0,16,27)  SampleTime=2.26757369614512e-05  VectorParamsAs1DForOutWhenUnconnected=off
  wires:
  Data_Sorter_Switch/1 -> Delay1/1
  Delay1/1 -> High_Data/1
  Relational Operator2/1 -> Data_Sorter_Switch/2
  Signal1/1 -> Relational Operator2/1, Data_Sorter_Switch/3, Data_Sorter_Switch/1
  Signal2/1 -> Relational Operator2/2

== system gm_final_heart_sym2_level4_hdl/DWT_Sym2_Level4/Threshold_Estimator/Median2/Data_Sorter24 ==
  Signal1 : Inport  OutDataTypeStr=fixdt(0, 16, 27)  PortDimensions=1  SampleTime=2.26757369614512e-05
  Signal2 : Inport  Port=2  OutDataTypeStr=fixdt(0, 16, 27)  PortDimensions=1  SampleTime=2.26757369614512e-05
  Data_Sorter_Switch : Switch  Criteria=u2 ~= 0  Threshold=double(0)  OutDataTypeStr=fixdt(0, 16, 27)  SampleTime=2.26757369614512e-05
  Data_Sorter_Switch1 : Switch  Threshold=double(1)  OutDataTypeStr=fixdt(0, 16, 27)  SampleTime=2.26757369614512e-05
  Delay1 : Delay  DelayLength=double(1)  InitialCondition=0  SampleTime=2.26757369614512e-05
  Delay2 : Delay  DelayLength=double(1)  InitialCondition=0  SampleTime=2.26757369614512e-05
  Relational Operator2 : RelationalOperator  Operator=<  OutDataTypeStr=boolean  SampleTime=2.26757369614512e-05  RndMeth=Nearest
  High_Data : Outport  OutDataTypeStr=fixdt(0,16,27)  SampleTime=2.26757369614512e-05  VectorParamsAs1DForOutWhenUnconnected=off
  Low_Data : Outport  Port=2  OutDataTypeStr=fixdt(0,16,27)  SampleTime=2.26757369614512e-05  VectorParamsAs1DForOutWhenUnconnected=off
  wires:
  Data_Sorter_Switch/1 -> Delay1/1
  Data_Sorter_Switch1/1 -> Delay2/1
  Delay1/1 -> High_Data/1
  Delay2/1 -> Low_Data/1
  Relational Operator2/1 -> Data_Sorter_Switch1/2, Data_Sorter_Switch/2
  Signal1/1 -> Relational Operator2/1, Data_Sorter_Switch/3, Data_Sorter_Switch/1
  Signal2/1 -> Relational Operator2/2, Data_Sorter_Switch1/3, Data_Sorter_Switch1/1

== system gm_final_heart_sym2_level4_hdl/DWT_Sym2_Level4/Threshold_Estimator/Median2/Data_Sorter3 ==
  Signal1 : Inport  OutDataTypeStr=fixdt(0, 16, 27)  PortDimensions=1  SampleTime=2.26757369614512e-05
  Signal2 : Inport  Port=2  OutDataTypeStr=fixdt(0, 16, 27)  PortDimensions=1  SampleTime=2.26757369614512e-05
  Data_Sorter_Switch : Switch  Criteria=u2 ~= 0  Threshold=double(0)  OutDataTypeStr=fixdt(0, 16, 27)  SampleTime=2.26757369614512e-05
  Data_Sorter_Switch1 : Switch  Threshold=double(1)  OutDataTypeStr=fixdt(0, 16, 27)  SampleTime=2.26757369614512e-05
  Delay1 : Delay  DelayLength=double(1)  InitialCondition=0  SampleTime=2.26757369614512e-05
  Delay2 : Delay  DelayLength=double(1)  InitialCondition=0  SampleTime=2.26757369614512e-05
  Relational Operator2 : RelationalOperator  Operator=<  OutDataTypeStr=boolean  SampleTime=2.26757369614512e-05  RndMeth=Nearest
  High_Data : Outport  OutDataTypeStr=fixdt(0,16,27)  SampleTime=2.26757369614512e-05  VectorParamsAs1DForOutWhenUnconnected=off
  Low_Data : Outport  Port=2  OutDataTypeStr=fixdt(0,16,27)  SampleTime=2.26757369614512e-05  VectorParamsAs1DForOutWhenUnconnected=off
  wires:
  Data_Sorter_Switch/1 -> Delay1/1
  Data_Sorter_Switch1/1 -> Delay2/1
  Delay1/1 -> High_Data/1
  Delay2/1 -> Low_Data/1
  Relational Operator2/1 -> Data_Sorter_Switch1/2, Data_Sorter_Switch/2
  Signal1/1 -> Relational Operator2/1, Data_Sorter_Switch/3, Data_Sorter_Switch/1
  Signal2/1 -> Relational Operator2/2, Data_Sorter_Switch1/3, Data_Sorter_Switch1/1

== system gm_final_heart_sym2_level4_hdl/DWT_Sym2_Level4/Threshold_Estimator/Median2/Data_Sorter4 ==
  Signal1 : Inport  OutDataTypeStr=fixdt(0, 16, 27)  PortDimensions=1  SampleTime=2.26757369614512e-05
  Signal2 : Inport  Port=2  OutDataTypeStr=fixdt(0, 16, 27)  PortDimensions=1  SampleTime=2.26757369614512e-05
  Data_Sorter_Switch : Switch  Criteria=u2 ~= 0  Threshold=double(0)  OutDataTypeStr=fixdt(0, 16, 27)  SampleTime=2.26757369614512e-05
  Data_Sorter_Switch1 : Switch  Threshold=double(1)  OutDataTypeStr=fixdt(0, 16, 27)  SampleTime=2.26757369614512e-05
  Delay1 : Delay  DelayLength=double(1)  InitialCondition=0  SampleTime=2.26757369614512e-05
  Delay2 : Delay  DelayLength=double(1)  InitialCondition=0  SampleTime=2.26757369614512e-05
  Relational Operator2 : RelationalOperator  Operator=<  OutDataTypeStr=boolean  SampleTime=2.26757369614512e-05  RndMeth=Nearest
  High_Data : Outport  OutDataTypeStr=fixdt(0,16,27)  SampleTime=2.26757369614512e-05  VectorParamsAs1DForOutWhenUnconnected=off
  Low_Data : Outport  Port=2  OutDataTypeStr=fixdt(0,16,27)  SampleTime=2.26757369614512e-05  VectorParamsAs1DForOutWhenUnconnected=off
  wires:
  Data_Sorter_Switch/1 -> Delay1/1
  Data_Sorter_Switch1/1 -> Delay2/1
  Delay1/1 -> High_Data/1
  Delay2/1 -> Low_Data/1
  Relational Operator2/1 -> Data_Sorter_Switch1/2, Data_Sorter_Switch/2
  Signal1/1 -> Relational Operator2/1, Data_Sorter_Switch/3, Data_Sorter_Switch/1
  Signal2/1 -> Relational Operator2/2, Data_Sorter_Switch1/3, Data_Sorter_Switch1/1

== system gm_final_heart_sym2_level4_hdl/DWT_Sym2_Level4/Threshold_Estimator/Median2/Data_Sorter5 ==
  Signal1 : Inport  OutDataTypeStr=fixdt(0, 16, 27)  PortDimensions=1  SampleTime=2.26757369614512e-05
  Signal2 : Inport  Port=2  OutDataTypeStr=fixdt(0, 16, 27)  PortDimensions=1  SampleTime=2.26757369614512e-05
  Data_Sorter_Switch : Switch  Criteria=u2 ~= 0  Threshold=double(0)  OutDataTypeStr=fixdt(0, 16, 27)  SampleTime=2.26757369614512e-05
  Data_Sorter_Switch1 : Switch  Threshold=double(1)  OutDataTypeStr=fixdt(0, 16, 27)  SampleTime=2.26757369614512e-05
  Delay1 : Delay  DelayLength=double(1)  InitialCondition=0  SampleTime=2.26757369614512e-05
  Delay2 : Delay  DelayLength=double(1)  InitialCondition=0  SampleTime=2.26757369614512e-05
  Relational Operator2 : RelationalOperator  Operator=<  OutDataTypeStr=boolean  SampleTime=2.26757369614512e-05  RndMeth=Nearest
  High_Data : Outport  OutDataTypeStr=fixdt(0,16,27)  SampleTime=2.26757369614512e-05  VectorParamsAs1DForOutWhenUnconnected=off
  Low_Data : Outport  Port=2  OutDataTypeStr=fixdt(0,16,27)  SampleTime=2.26757369614512e-05  VectorParamsAs1DForOutWhenUnconnected=off
  wires:
  Data_Sorter_Switch/1 -> Delay1/1
  Data_Sorter_Switch1/1 -> Delay2/1
  Delay1/1 -> High_Data/1
  Delay2/1 -> Low_Data/1
  Relational Operator2/1 -> Data_Sorter_Switch1/2, Data_Sorter_Switch/2
  Signal1/1 -> Relational Operator2/1, Data_Sorter_Switch/3, Data_Sorter_Switch/1
  Signal2/1 -> Relational Operator2/2, Data_Sorter_Switch1/3, Data_Sorter_Switch1/1

== system gm_final_heart_sym2_level4_hdl/DWT_Sym2_Level4/Threshold_Estimator/Median2/Data_Sorter6 ==
  Signal1 : Inport  OutDataTypeStr=fixdt(0, 16, 27)  PortDimensions=1  SampleTime=2.26757369614512e-05
  Signal2 : Inport  Port=2  OutDataTypeStr=fixdt(0, 16, 27)  PortDimensions=1  SampleTime=2.26757369614512e-05
  Data_Sorter_Switch : Switch  Criteria=u2 ~= 0  Threshold=double(0)  OutDataTypeStr=fixdt(0, 16, 27)  SampleTime=2.26757369614512e-05
  Data_Sorter_Switch1 : Switch  Threshold=double(1)  OutDataTypeStr=fixdt(0, 16, 27)  SampleTime=2.26757369614512e-05
  Delay1 : Delay  DelayLength=double(1)  InitialCondition=0  SampleTime=2.26757369614512e-05
  Delay2 : Delay  DelayLength=double(1)  InitialCondition=0  SampleTime=2.26757369614512e-05
  Relational Operator2 : RelationalOperator  Operator=<  OutDataTypeStr=boolean  SampleTime=2.26757369614512e-05  RndMeth=Nearest
  High_Data : Outport  OutDataTypeStr=fixdt(0,16,27)  SampleTime=2.26757369614512e-05  VectorParamsAs1DForOutWhenUnconnected=off
  Low_Data : Outport  Port=2  OutDataTypeStr=fixdt(0,16,27)  SampleTime=2.26757369614512e-05  VectorParamsAs1DForOutWhenUnconnected=off
  wires:
  Data_Sorter_Switch/1 -> Delay1/1
  Data_Sorter_Switch1/1 -> Delay2/1
  Delay1/1 -> High_Data/1
  Delay2/1 -> Low_Data/1
  Relational Operator2/1 -> Data_Sorter_Switch1/2, Data_Sorter_Switch/2
  Signal1/1 -> Relational Operator2/1, Data_Sorter_Switch/3, Data_Sorter_Switch/1
  Signal2/1 -> Relational Operator2/2, Data_Sorter_Switch1/3, Data_Sorter_Switch1/1

== system gm_final_heart_sym2_level4_hdl/DWT_Sym2_Level4/Threshold_Estimator/Median2/Data_Sorter7 ==
  Signal1 : Inport  OutDataTypeStr=fixdt(0, 16, 27)  PortDimensions=1  SampleTime=2.26757369614512e-05
  Signal2 : Inport  Port=2  OutDataTypeStr=fixdt(0, 16, 27)  PortDimensions=1  SampleTime=2.26757369614512e-05
  Data_Sorter_Switch : Switch  Criteria=u2 ~= 0  Threshold=double(0)  OutDataTypeStr=fixdt(0, 16, 27)  SampleTime=2.26757369614512e-05
  Data_Sorter_Switch1 : Switch  Threshold=double(1)  OutDataTypeStr=fixdt(0, 16, 27)  SampleTime=2.26757369614512e-05
  Delay1 : Delay  DelayLength=double(1)  InitialCondition=0  SampleTime=2.26757369614512e-05
  Delay2 : Delay  DelayLength=double(1)  InitialCondition=0  SampleTime=2.26757369614512e-05
  Relational Operator2 : RelationalOperator  Operator=<  OutDataTypeStr=boolean  SampleTime=2.26757369614512e-05  RndMeth=Nearest
  High_Data : Outport  OutDataTypeStr=fixdt(0,16,27)  SampleTime=2.26757369614512e-05  VectorParamsAs1DForOutWhenUnconnected=off
  Low_Data : Outport  Port=2  OutDataTypeStr=fixdt(0,16,27)  SampleTime=2.26757369614512e-05  VectorParamsAs1DForOutWhenUnconnected=off
  wires:
  Data_Sorter_Switch/1 -> Delay1/1
  Data_Sorter_Switch1/1 -> Delay2/1
  Delay1/1 -> High_Data/1
  Delay2/1 -> Low_Data/1
  Relational Operator2/1 -> Data_Sorter_Switch1/2, Data_Sorter_Switch/2
  Signal1/1 -> Relational Operator2/1, Data_Sorter_Switch/3, Data_Sorter_Switch/1
  Signal2/1 -> Relational Operator2/2, Data_Sorter_Switch1/3, Data_Sorter_Switch1/1

== system gm_final_heart_sym2_level4_hdl/DWT_Sym2_Level4/Threshold_Estimator/Median2/Data_Sorter8 ==
  Signal1 : Inport  OutDataTypeStr=fixdt(0, 16, 27)  PortDimensions=1  SampleTime=2.26757369614512e-05
  Signal2 : Inport  Port=2  OutDataTypeStr=fixdt(0, 16, 27)  PortDimensions=1  SampleTime=2.26757369614512e-05
  Data_Sorter_Switch : Switch  Criteria=u2 ~= 0  Threshold=double(0)  OutDataTypeStr=fixdt(0, 16, 27)  SampleTime=2.26757369614512e-05
  Data_Sorter_Switch1 : Switch  Threshold=double(1)  OutDataTypeStr=fixdt(0, 16, 27)  SampleTime=2.26757369614512e-05
  Delay1 : Delay  DelayLength=double(1)  InitialCondition=0  SampleTime=2.26757369614512e-05
  Delay2 : Delay  DelayLength=double(1)  InitialCondition=0  SampleTime=2.26757369614512e-05
  Relational Operator2 : RelationalOperator  Operator=<  OutDataTypeStr=boolean  SampleTime=2.26757369614512e-05  RndMeth=Nearest
  High_Data : Outport  OutDataTypeStr=fixdt(0,16,27)  SampleTime=2.26757369614512e-05  VectorParamsAs1DForOutWhenUnconnected=off
  Low_Data : Outport  Port=2  OutDataTypeStr=fixdt(0,16,27)  SampleTime=2.26757369614512e-05  VectorParamsAs1DForOutWhenUnconnected=off
  wires:
  Data_Sorter_Switch/1 -> Delay1/1
  Data_Sorter_Switch1/1 -> Delay2/1
  Delay1/1 -> High_Data/1
  Delay2/1 -> Low_Data/1
  Relational Operator2/1 -> Data_Sorter_Switch1/2, Data_Sorter_Switch/2
  Signal1/1 -> Relational Operator2/1, Data_Sorter_Switch/3, Data_Sorter_Switch/1
  Signal2/1 -> Relational Operator2/2, Data_Sorter_Switch1/3, Data_Sorter_Switch1/1

== system gm_final_heart_sym2_level4_hdl/DWT_Sym2_Level4/Threshold_Estimator/Median2/Data_Sorter9 ==
  Signal1 : Inport  OutDataTypeStr=fixdt(0, 16, 27)  PortDimensions=1  SampleTime=2.26757369614512e-05
  Signal2 : Inport  Port=2  OutDataTypeStr=fixdt(0, 16, 27)  PortDimensions=1  SampleTime=2.26757369614512e-05
  Data_Sorter_Switch : Switch  Criteria=u2 ~= 0  Threshold=double(0)  OutDataTypeStr=fixdt(0, 16, 27)  SampleTime=2.26757369614512e-05
  Data_Sorter_Switch1 : Switch  Threshold=double(1)  OutDataTypeStr=fixdt(0, 16, 27)  SampleTime=2.26757369614512e-05
  Delay1 : Delay  DelayLength=double(1)  InitialCondition=0  SampleTime=2.26757369614512e-05
  Delay2 : Delay  DelayLength=double(1)  InitialCondition=0  SampleTime=2.26757369614512e-05
  Relational Operator2 : RelationalOperator  Operator=<  OutDataTypeStr=boolean  SampleTime=2.26757369614512e-05  RndMeth=Nearest
  High_Data : Outport  OutDataTypeStr=fixdt(0,16,27)  SampleTime=2.26757369614512e-05  VectorParamsAs1DForOutWhenUnconnected=off
  Low_Data : Outport  Port=2  OutDataTypeStr=fixdt(0,16,27)  SampleTime=2.26757369614512e-05  VectorParamsAs1DForOutWhenUnconnected=off
  wires:
  Data_Sorter_Switch/1 -> Delay1/1
  Data_Sorter_Switch1/1 -> Delay2/1
  Delay1/1 -> High_Data/1
  Delay2/1 -> Low_Data/1
  Relational Operator2/1 -> Data_Sorter_Switch1/2, Data_Sorter_Switch/2
  Signal1/1 -> Relational Operator2/1, Data_Sorter_Switch/3, Data_Sorter_Switch/1
  Signal2/1 -> Relational Operator2/2, Data_Sorter_Switch1/3, Data_Sorter_Switch1/1
